simulink model "BP2_in"  (R2015a)
settings: Solver=ode3  SolverMode=SingleTasking  StartTime=0.0  StopTime=6e-3  FixedStep=Ts  MaxStep=3.90625e-06  RelTol=1e-3  AbsTol=1e-3
undefined symbols (not defined in the file): b, b2, b3, Cf, clock, delta, k, noise1, Temp, Ts, Vref
CloseFcn:
  | ;slview('closediagram',bdroot);
settings Model: Creator=thaodang  LastModifiedBy=thaodang
settings DataIOCC: LimitDataPoints=off  SignalLoggingSaveFormat=ModelDataLogs  SaveOutput=off  SaveTime=off
settings OptimizationCC: BlockReduction=off  BooleanDataType=off
settings DebuggingCC: SaveWithParameterizedLinksMsg=none  UnderspecifiedInitializationDetection=Classic  MergeDetectMultiDrivingBlocksExec=none  SignalResolutionControl=TryResolveAllWithWarning  MultiTaskDSMMsg=warning  MultiTaskCondExecSysMsg=none
settings HardwareCC: TargetUnknown=on
settings RTWCC: TemplateMakefile=grt.tmf
settings GRTTargetCC: CombineOutputUpdateFcns=off  GRTInterface=on

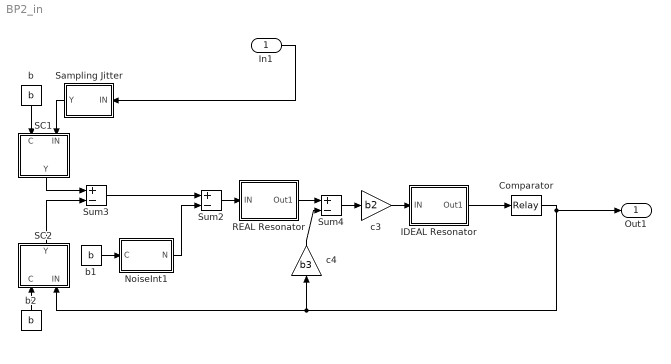
== system BP2_in ==
  In1 : Inport
  Comparator : Relay  OnOutputValue=Vref  OffOutputValue=-Vref
  IDEAL Resonator : Subsystem  mask(Integrator){Ts=Ts}
      mask prompts: Ts "Sample Time:"
      mask help: Ideal discrete resonator with delay.
      mask Help:
      | Parameters:
      | Ts:       Sample time
      mask Display: dpoly([0 0 -1], [1 0 1], 'z-')
  NoiseInt1 : Subsystem  mask(OpAmp Noise){seed=sum(clock)^1/111, Ts=Ts, noise=noise1}
      mask prompts: seed "Random Number Seed:"; Ts "Sample Time:"; noise "Op-amp Noise Std. Dev.:"
      mask Display: disp('OpNoise')
  REAL Resonator : Subsystem  mask(Integrator){Ts=2.3364e-08, alfa=0.9986, Amax=2, sr=280000000, GBW=250000000}
      mask prompts: Ts "Sample Time:"; alfa "Finite Gain:"; Amax "Saturation:"; sr "Slew Rate:"; GBW "Gain-Bandwidth"
      mask help:
      | Real discrete integrator with delay.
      | Models op-amp saturation and slew rate.
      mask Help:
      | Parameters:
      | Ts:       Sample time
      | G:         Finite op-amp gain (ideal op-amp G=1)
      | Amax:  Saturation value
      | sr:       slew rate in V/s
      mask Display: dpoly([0 0 -1], [1 0 1], 'z-')
  SC1 : Subsystem  mask(kT/C Noise){Ts=Ts, Ci=Cf, Temp=Temp, k=k, seed=sum(clock)}
      mask prompts: Ts "Sample Time:"; Ci "Integrating Capacitance:"; Temp "Absolute Temperature:"; k "Boltzman Constant:"; seed "Random Number Seed:"
      mask help:
      | Models the kT/Cs noise of a switched capacitance Cs.
      | IN input: the input signal line
      | C input:   accepts the coefficient WITH SIGN (Cs/Ci)
      mask Help:
      | Block parameters:
      | Ts:        Sample time
      | Ci:        Integrating Capacitance
      | Temp:   Absolute Temperature in Kelvin
      | k:         Boltzmann Constant
      | seed:    Initial seed for random number generator
      | Outputs the noisy signal.
      mask Display: disp('kT/C')
  SC2 : Subsystem  mask(kT/C Noise){Ts=Ts, Ci=Cf, Temp=Temp, k=k, seed=2.11*sum(clock)}
      mask prompts: Ts "Sample Time:"; Ci "Integrating Capacitance:"; Temp "Absolute Temperature:"; k "Boltzman Constant:"; seed "Random Number Seed:"
      mask help:
      | Models the kT/Cs noise of a switched capacitance Cs.
      | IN input: the input signal line
      | C input:   accepts the coefficient WITH SIGN (Cs/Ci)
      mask Help:
      | Block parameters:
      | Ts:        Sample time
      | Ci:        Integrating Capacitance
      | Temp:   Absolute Temperature in Kelvin
      | k:         Boltzmann Constant
      | seed:    Initial seed for random number generator
      | Outputs the noisy signal.
      mask Display: disp('kT/C')
  Sampling Jitter : Subsystem  mask(Jitter){Ts=Ts, delta=delta, seed=(sum(clock))^3.33}
      mask prompts: Ts "Sample Time:"; delta "Sampling Jitter:"; seed "Random Number Seed:"
      mask help:
      | Models the kT/Cs noise of a switched capacitance Cs.
      | IN input: the input signal line
      | C input:   accepts the coefficient WITH SIGN (Cs/Ci)
      mask Help:
      | Block parameters:
      | Ts:        Sample time
      | Ci:        Integrating Capacitance
      | Temp:   Absolute Temperature in Kelvin
      | k:         Boltzmann Constant
      | seed:    Initial seed for random number generator
      | Outputs the noisy signal.
      mask Display: disp('Jitter')
  Sum2 : Sum  Inputs=+-  SaturateOnIntegerOverflow=on  InputSameDT=on  OutDataTypeStr=Inherit: Same as first input
  Sum3 : Sum  Inputs=+-  SaturateOnIntegerOverflow=on  InputSameDT=on  OutDataTypeStr=Inherit: Same as first input
  Sum4 : Sum  Inputs=+-  SaturateOnIntegerOverflow=on  InputSameDT=on  OutDataTypeStr=Inherit: Same as first input
  b : Constant  Value=b
  b1 : Constant  Value=b
  b2 : Constant  Value=b
  c3 : Gain  Gain=b2  SaturateOnIntegerOverflow=on  OutDataTypeStr=Inherit: Same as input  ParamDataTypeStr=Inherit: Same as input
  c4 : Gain  Gain=b3  SaturateOnIntegerOverflow=on  OutDataTypeStr=Inherit: Same as input  ParamDataTypeStr=Inherit: Same as input
  Out1 : Outport
  wires:
  Sum2/1 -> REAL Resonator/1(IN)
  Sum4/1 -> c3/1
  c3/1 -> IDEAL Resonator/1(IN)
  NoiseInt1/1(N) -> Sum2/2
  b1/1 -> NoiseInt1/1(C)
  Sum3/1 -> Sum2/1
  SC1/1(Y) -> Sum3/1
  b/1 -> SC1/1(C)
  SC2/1(Y) -> Sum3/2
  Sampling Jitter/1(Y) -> SC1/2(IN)
  b2/1 -> SC2/1(C)
  REAL Resonator/1(Out1) -> Sum4/1
  Comparator/1 -> Out1/1, SC2/2(IN), c4/1
  IDEAL Resonator/1(Out1) -> Comparator/1
  c4/1 -> Sum4/2
  In1/1 -> Sampling Jitter/1(IN)

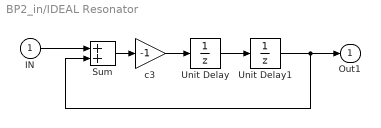
== system BP2_in/IDEAL Resonator ==
  IN : Inport
  Sum : Sum  SaturateOnIntegerOverflow=on  InputSameDT=on  OutDataTypeStr=Inherit: Same as first input
  Unit Delay : UnitDelay  InitialCondition=1  SampleTime=-1
  Unit Delay1 : UnitDelay  InitialCondition=1  SampleTime=-1
  c3 : Gain  Gain=-1  SaturateOnIntegerOverflow=on  OutDataTypeStr=Inherit: Same as input  ParamDataTypeStr=Inherit: Same as input
  Out1 : Outport
  wires:
  IN/1 -> Sum/1
  Unit Delay/1 -> Unit Delay1/1
  Unit Delay1/1 -> Out1/1, Sum/2
  Sum/1 -> c3/1
  c3/1 -> Unit Delay/1

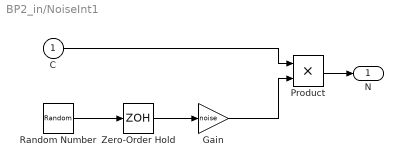
== system BP2_in/NoiseInt1 ==
  C : Inport
  Gain : Gain  Gain=noise  SaturateOnIntegerOverflow=on  OutDataTypeStr=Inherit: Same as input  ParamDataTypeStr=Inherit: Same as input
  Product : Product  SaturateOnIntegerOverflow=on  RndMeth=Zero  InputSameDT=on  OutDataTypeStr=Inherit: Same as first input
  Random Number : RandomNumber  Seed=seed  SampleTime=Ts
  Zero-Order Hold : ZeroOrderHold  SampleTime=Ts
  N : Outport  InitialOutput=0
  wires:
  Random Number/1 -> Zero-Order Hold/1
  Zero-Order Hold/1 -> Gain/1
  Product/1 -> N/1
  Gain/1 -> Product/2
  C/1 -> Product/1

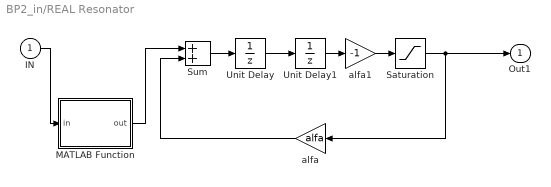
== system BP2_in/REAL Resonator ==
  IN : Inport
  MATLAB Function : MATLAB Function  TreatAsAtomicUnit=on
  Saturation : Saturate  UpperLimit=Amax  LowerLimit=-Amax
  Sum : Sum  SaturateOnIntegerOverflow=on  InputSameDT=on  OutDataTypeStr=Inherit: Same as first input
  Unit Delay : UnitDelay  InitialCondition=1  SampleTime=-1
  Unit Delay1 : UnitDelay  InitialCondition=1  SampleTime=-1
  alfa : Gain  Gain=alfa  SaturateOnIntegerOverflow=on  OutDataTypeStr=Inherit: Same as input  ParamDataTypeStr=Inherit: Same as input
  alfa1 : Gain  Gain=-1  SaturateOnIntegerOverflow=on  OutDataTypeStr=Inherit: Same as input  ParamDataTypeStr=Inherit: Same as input
  Out1 : Outport
  wires:
  Sum/1 -> Unit Delay/1
  Saturation/1 -> Out1/1, alfa/1
  IN/1 -> MATLAB Function/1(in)
  MATLAB Function/1(out) -> Sum/1
  alfa/1 -> Sum/2
  Unit Delay/1 -> Unit Delay1/1
  Unit Delay1/1 -> alfa1/1
  alfa1/1 -> Saturation/1

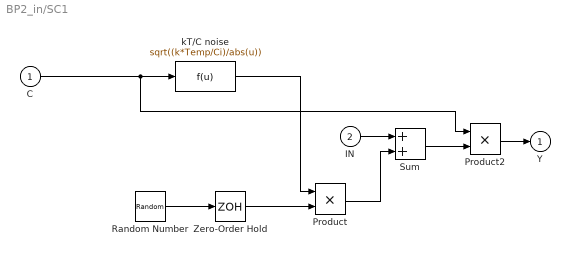
== system BP2_in/SC1 ==
  C : Inport
  IN : Inport  Port=2
  Product : Product  SaturateOnIntegerOverflow=on  RndMeth=Zero  InputSameDT=on  OutDataTypeStr=Inherit: Same as first input
  Product2 : Product  SaturateOnIntegerOverflow=on  RndMeth=Zero  InputSameDT=on  OutDataTypeStr=Inherit: Same as first input
  Random Number : RandomNumber  Seed=seed  SampleTime=Ts
  Sum : Sum  SaturateOnIntegerOverflow=on  InputSameDT=on  OutDataTypeStr=Inherit: Same as first input
  Zero-Order Hold : ZeroOrderHold  SampleTime=Ts
  kT/C noise : Fcn  Expr=sqrt((k*Temp/Ci)/abs(u))
  Y : Outport  InitialOutput=0
  wires:
  Random Number/1 -> Zero-Order Hold/1
  C/1 -> Product2/1, kT/C noise/1
  Zero-Order Hold/1 -> Product/2
  kT/C noise/1 -> Product/1
  Sum/1 -> Product2/2
  IN/1 -> Sum/1
  Product2/1 -> Y/1
  Product/1 -> Sum/2

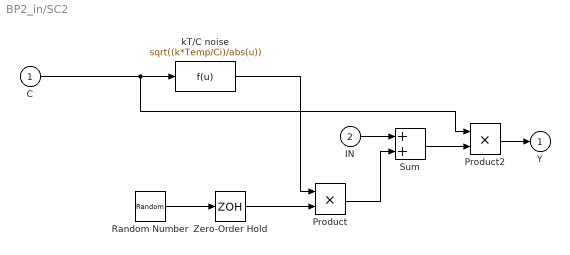
== system BP2_in/SC2 ==
  C : Inport
  IN : Inport  Port=2
  Product : Product  SaturateOnIntegerOverflow=on  RndMeth=Zero  InputSameDT=on  OutDataTypeStr=Inherit: Same as first input
  Product2 : Product  SaturateOnIntegerOverflow=on  RndMeth=Zero  InputSameDT=on  OutDataTypeStr=Inherit: Same as first input
  Random Number : RandomNumber  Seed=seed  SampleTime=Ts
  Sum : Sum  SaturateOnIntegerOverflow=on  InputSameDT=on  OutDataTypeStr=Inherit: Same as first input
  Zero-Order Hold : ZeroOrderHold  SampleTime=Ts
  kT/C noise : Fcn  Expr=sqrt((k*Temp/Ci)/abs(u))
  Y : Outport  InitialOutput=0
  wires:
  Random Number/1 -> Zero-Order Hold/1
  C/1 -> Product2/1, kT/C noise/1
  Zero-Order Hold/1 -> Product/2
  kT/C noise/1 -> Product/1
  Sum/1 -> Product2/2
  IN/1 -> Sum/1
  Product2/1 -> Y/1
  Product/1 -> Sum/2

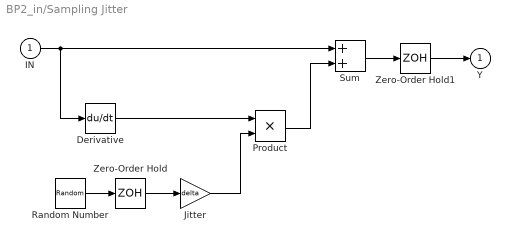
== system BP2_in/Sampling Jitter ==
  IN : Inport
  Derivative : Derivative
  Jitter : Gain  Gain=delta  SaturateOnIntegerOverflow=on  OutDataTypeStr=Inherit: Same as input  ParamDataTypeStr=Inherit: Same as input
  Product : Product  SaturateOnIntegerOverflow=on  RndMeth=Zero  InputSameDT=on  OutDataTypeStr=Inherit: Same as first input
  Random Number : RandomNumber  Seed=seed  SampleTime=Ts
  Sum : Sum  SaturateOnIntegerOverflow=on  InputSameDT=on  OutDataTypeStr=Inherit: Same as first input
  Zero-Order Hold : ZeroOrderHold  SampleTime=Ts
  Zero-Order Hold1 : ZeroOrderHold  SampleTime=Ts
  Y : Outport  InitialOutput=0
  wires:
  IN/1 -> Sum/1, Derivative/1
  Random Number/1 -> Zero-Order Hold/1
  Derivative/1 -> Product/1
  Zero-Order Hold/1 -> Jitter/1
  Jitter/1 -> Product/2
  Product/1 -> Sum/2
  Sum/1 -> Zero-Order Hold1/1
  Zero-Order Hold1/1 -> Y/1

== matlab function BP2_in/REAL Resonator/MATLAB Function ==
  data: in input; out output
function out = slew(in)
% 
% Models the op-amp slew rate for a discrete time integrator
%
% in:   input signal amplitude
% alfa: effect of finite gain (ideal op-amp alfa=1)
% sr:   slew rate in V/s
% GBW:  gain-bandwidth product of the integrator in Hz
% Ts:   sample time
%
% out:  output signal amplitude

%%%%%%%

% ************************************************************************
% Variabili globali
% ************************************************************************
bw=200e3;				% Base-band
R=107;					% 42.8 MHz sampling rate
% R=50;					% 20.0 MHz sampling rate
Fs=R*2*bw;				% Oversampling frequency
Ts=1/Fs;
N=65536;				% Samples number
nper=4;
Fin=(Fs/4)+ nper*Fs/N;			% Input signal frequency (Fin=(Fs/4)+ nper*Fs/N)
Ampl=0.5-pi/256;		% Input signal amplitude [V]
Ntransient=0;
%
% kT/C noise and op-amp non-idealities
%
%echo on;
k=1.38e-23;				% Boltzmann Constant
Temp=300;				% Absolute Temperature in Kelvin
% Temp=0;				% Absolute Temperature in Kelvin
Cf=4e-12;				% Integrating Capacitance of the first integrator
alfa=(711-1)/711;		% A=Op-amp finite gain (alfa=(A-1)/A -> ideal op-amp alfa=1)
% alfa=1;
Amax=2;					% Op-amp saturation value [V]
% Amax=10000;					% Op-amp saturation value [V]
sr=280e6;				% Op-amp slew rate [V/s]
% sr=280e10;				% Op-amp slew rate [V/s]
GBW=250e6;				% Op-amp GBW [Hz]
% GBW=250e10;				% Op-amp GBW [Hz]
noise1=4.39e-3;			% 1st int. output noise std. dev. [Vrms]
% noise1=0;
delta=0.1e-9;				% Random Sampling jitter (std. dev.) [s] (Boser, Wooley JSSC Dec. 88)
% delta=0;
%echo off;
% Modulator coefficients

%echo on;
b=0.125;		% 1/8 gain of the first stage
b2=0.125;	% 1/8 gain of the second stage
b3=0.25;		% 1/4 additional gain of the second feedback loop
Vref=1;
%echo off;

finrad=Fin*2*pi;		% Input signal frequency in radians



%%%%%%%

tau=1/(2*pi*GBW);  % Time constant of the integrator
Tmax = Ts/2;

slope=alfa*abs(in)/tau;

if slope > sr			% Op-amp in slewing
	
	tsl = abs(in)*alfa/sr - tau;  % Slewing time
	
	if tsl >= Tmax
		error = abs(in) - sr*Tmax;
	else
		texp = Tmax - tsl;
		error = abs(in)*(1-alfa) + (alfa*abs(in) - sr*tsl) * exp(-texp/tau);
	end
	
else					% Op-amp in linear region
	texp = Tmax;
	error = abs(in)*(1-alfa) + alfa*abs(in) * exp(-texp/tau);
end

out = in - sign(in)*error;
